simulink model "control_3quads_attached_LIEKF"  (R2019a)
settings: Solver=FixedStepAuto  StartTime=0.0  StopTime=60  FixedStep=0.025  RelTol=1e-3  EnableMultiTasking=on
InitFcn:
  | global clientID;
  | clientID=-1;
  | 
  | global R_t;
  | global A_t;
  | global P_t;
  | global H;
  | global Q;
  | global N;
  | 
  | R_t=eye(3);
  | A_t=eye(3)*0;
  | P_t=eye(3)*0.001;
  | H=eye(3);
  | Q=eye(3);
  | N=eye(3);
values from neighbouring files (symbols this model uses):
  X = reshape(X, size(A_t))    [RiccatiCov.m]
undefined symbols (not defined in the file or in its folder): Y, Z
libraries: robotlib x10, dspindex x3, simulink_extras x1
settings Model: Creator=Kleber Cabral  LastModifiedBy=Kleber Cabral
settings SolverCC: AutoInsertRateTranBlk=on
settings DataIOCC: SaveFormat=Array  ReturnWorkspaceOutputs=off
settings OptimizationCC: LifeSpan=inf
settings DebuggingCC: SolverPrmCheckMsg=warning  SFUnexpectedBacktrackingDiag=warning  SFNoUnconditionalDefaultTransitionDiag=warning  ArithmeticOperatorsInVariantConditions=warning
settings HardwareCC: ProdBitPerPointer=32  ProdBitPerSizeT=32  ProdBitPerPtrDiffT=32  ProdLargestAtomicFloat=None  ProdIntDivRoundTo=Undefined  ProdEndianess=Unspecified  ProdWordSize=32  ProdHWDeviceType=32-bit Generic
settings ModelReferenceCC: PropagateSignalLabelsOutOfModel=off
settings SFSimCC: SimUseLocalCustomCode=off
settings RTWCC: RTWUseLocalCustomCode=off
settings CodeAppCC: StateflowObjectComments=on
settings GRTTargetCC: TargetLangStandard=C89/C90 (ANSI)  GeneratePreprocessorConditionals=Disable all
settings ConfigComp: CovMetricSettings=dw  CovHtmlReporting=on  CovSaveCumulativeToWorkspaceVar=on  CovSaveSingleToWorkspaceVar=on  CovExternalEMLEnable=off  CovSFcnEnable=off

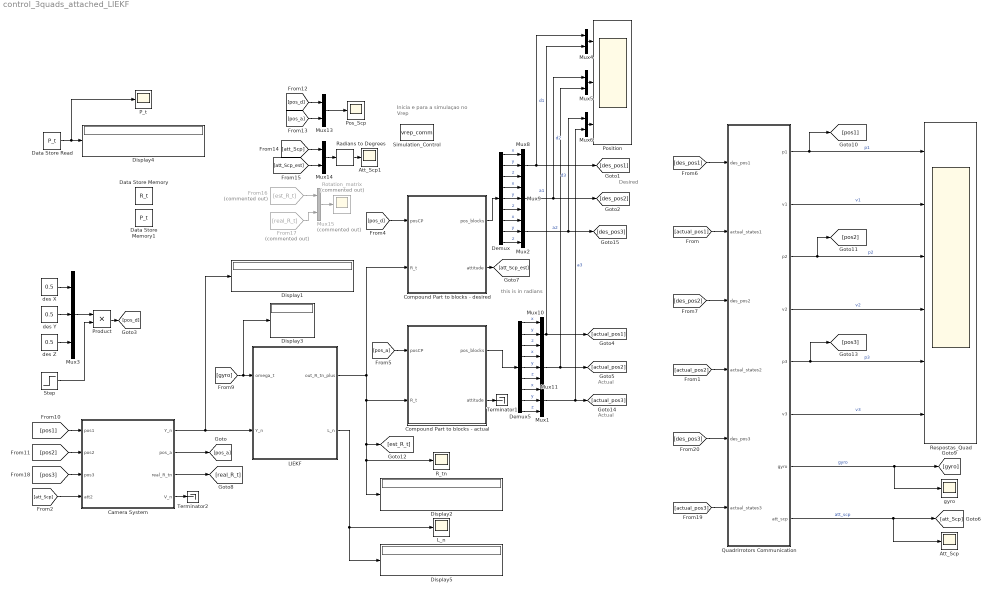
== system control_3quads_attached_LIEKF ==
  note: this is in radians
  note: Desired
  note: Inicia e para a simulaçao no Vrep
  note: Actual
  note: Actual
  Att_Scp : Scope
  Att_Scp1 : Scope
  Camera System : Subsystem
  Compound Part to blocks - actual : MATLAB Function  TreatAsAtomicUnit=on
  Compound Part to blocks - desired : MATLAB Function  TreatAsAtomicUnit=on
  Data Store Memory : DataStoreMemory  DataStoreName=R_t  ReadBeforeWriteMsg=warning  WriteAfterWriteMsg=warning  WriteAfterReadMsg=warning  InitialValue=eye(3)  ShowAdditionalParam=off  OutDataTypeStr=double
  Data Store Memory1 : DataStoreMemory  DataStoreName=P_t  ReadBeforeWriteMsg=warning  WriteAfterWriteMsg=warning  WriteAfterReadMsg=warning  InitialValue=eye(3)*0.001  ShowAdditionalParam=off  OutDataTypeStr=double
  Data Store Read : DataStoreRead  DataStoreName=P_t
  Demux : Demux  Outputs=9
  Demux5 : Demux  Outputs=9
  Display{1..5} (5 alike) : Display
      settings: Decimation=3
  From16 : From  Commented=on  GotoTag=est_R_t
  From17 : From  Commented=on  GotoTag=real_R_t
  LIEKF : MATLAB Function  TreatAsAtomicUnit=on
  L_n : Scope
  Mux{1..3,8..11} (7 alike) : Mux  Inputs=3
  Mux{4..6,13..14} (5 alike) : Mux  Inputs=2
  Mux15 : Mux  Commented=on  Inputs=2
  P_t : Scope
  Pos_Scp : Scope
  Position : Scope  NumInputPorts=3
  Product : Product
  Quadrirrotors Communication : Subsystem
  R_tn : Scope
  Radians to Degrees : simulink_extras/Transformations/Radians to Degrees
  Respostas_Quad : Scope  NumInputPorts=6
  Rotation_matrix : Scope  Commented=on
  Simulation_Control : S-Function  FunctionName=vrep_comm  SFunctionDeploymentMode=off  EnableBusSupport=off
  Step : Step  Time=5  SampleTime=0
  Terminator1 : Terminator
  Terminator2 : Terminator
  des X : Constant  Value=0.5
  des Y : Constant  Value=0.5
  des Z : Constant  Value=0.5
  gyro : Scope
  wires:
  des X/1 -> Mux3/1
  des Y/1 -> Mux3/2
  des Z/1 -> Mux3/3
  [pos1] -> Camera System/1(pos1)
  [pos2] -> Camera System/2(pos2)
  [pos_d] -> Compound Part to blocks - desired/1(posCP)
  Compound Part to blocks - desired/1(pos_blocks) -> Demux/1
  Compound Part to blocks - actual/1(pos_blocks) -> Demux5/1
  Mux8/1 -> Mux4/1, [des_pos1]  "d1"
  Demux/3 -> Mux8/3  "z"
  Demux/2 -> Mux8/2  "y"
  Demux/1 -> Mux8/1  "x"
  Mux9/1 -> Mux5/1, [des_pos2]  "d2"
  Demux/4 -> Mux9/1  "x"
  Demux/5 -> Mux9/2  "y"
  Demux/6 -> Mux9/3  "z"
  [des_pos1] -> Quadrirrotors Communication/1(des_pos1)
  [des_pos2] -> Quadrirrotors Communication/3(des_pos2)
  Mux11/1 -> Mux5/2, [actual_pos2]  "a2"
  Mux10/1 -> Mux4/2, [actual_pos1]  "a1"
  Demux5/1 -> Mux10/1  "x"
  Demux5/2 -> Mux10/2  "y"
  Demux5/3 -> Mux10/3  "z"
  Demux5/4 -> Mux11/1  "x"
  Demux5/5 -> Mux11/2  "y"
  Demux5/6 -> Mux11/3  "z"
  [actual_pos1] -> Quadrirrotors Communication/2(actual_states1)
  [actual_pos2] -> Quadrirrotors Communication/4(actual_states2)
  Camera System/2(pos_a) -> [pos_a]
  [att_Scp] -> Camera System/4(att2)
  Compound Part to blocks - desired/2(attitude) -> [att_Scp_est]
  Camera System/1(Y_n) -> Display1/1, LIEKF/2(Y_n)
  [gyro] -> Display3/1, LIEKF/1(omega_t)
  Compound Part to blocks - actual/2(attitude) -> Terminator1/1
  Data Store Read/1 -> P_t/1, Display4/1
  LIEKF/2(L_n) -> Display5/1, L_n/1
  LIEKF/1(out_R_tn_plus) -> Display2/1, R_tn/1, [est_R_t], Compound Part to blocks - actual/2(R_t), Compound Part to blocks - desired/2(R_t)
  [pos_a] -> Compound Part to blocks - actual/1(posCP)
  Mux3/1 -> Product/1
  Step/1 -> Product/2
  Product/1 -> [pos_d]
  Mux13/1 -> Pos_Scp/1
  [pos_d] -> Mux13/1
  [pos_a] -> Mux13/2
  [att_Scp] -> Mux14/1
  [att_Scp_est] -> Mux14/2
  Camera System/3(real_R_tn) -> [real_R_t]
  Camera System/4(V_n) -> Terminator2/1
  From16/1 -> Mux15/1
  From17/1 -> Mux15/2
  Mux15/1 -> Rotation_matrix/1
  Quadrirrotors Communication/1(p1) -> Respostas_Quad/1, [pos1]  "p1"
  Quadrirrotors Communication/2(v1) -> Respostas_Quad/2  "v1"
  Quadrirrotors Communication/3(p2) -> Respostas_Quad/3, [pos2]  "p2"
  Quadrirrotors Communication/4(v2) -> Respostas_Quad/4  "v2"
  Quadrirrotors Communication/7(gyro) -> gyro/1, [gyro]  "gyro"
  Quadrirrotors Communication/8(att_scp) -> Att_Scp/1, [att_Scp]  "att_scp"
  Quadrirrotors Communication/5(p3) -> Respostas_Quad/5, [pos3]  "p3"
  [pos3] -> Camera System/3(pos3)
  Quadrirrotors Communication/6(v3) -> Respostas_Quad/6  "v3"
  Demux5/9 -> Mux1/3  "z"
  Demux5/8 -> Mux1/2  "y"
  Demux5/7 -> Mux1/1  "x"
  Mux1/1 -> Mux6/2, [actual_pos3]  "a3"
  [actual_pos3] -> Quadrirrotors Communication/6(actual_states3)
  Demux/9 -> Mux2/3  "z"
  Demux/8 -> Mux2/2  "y"
  Demux/7 -> Mux2/1  "x"
  Mux2/1 -> Mux6/1, [des_pos3]  "d3"
  [des_pos3] -> Quadrirrotors Communication/5(des_pos3)
  Mux4/1 -> Position/1
  Mux5/1 -> Position/2
  Mux6/1 -> Position/3
  Radians to Degrees/1 -> Att_Scp1/1
  Mux14/1 -> Radians to Degrees/1

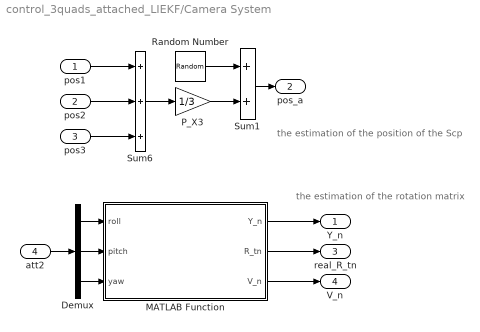
== system control_3quads_attached_LIEKF/Camera System ==
  note: the estimation of the rotation matrix
  note: the estimation of the position of the Scp
  pos1 : Inport
  pos2 : Inport  Port=2
  pos3 : Inport  Port=3
  att2 : Inport  Port=4
  Demux : Demux  Outputs=3
  MATLAB Function : MATLAB Function  TreatAsAtomicUnit=on
  P_X3 : Gain  Gain=1/3
  Random Number : RandomNumber  Variance=0.05
  Sum1 : Sum
  Sum6 : Sum  Inputs=+++
  Y_n : Outport
  pos_a : Outport  Port=2
  real_R_tn : Outport  Port=3
  V_n : Outport  Port=4
  wires:
  pos1/1 -> Sum6/1
  pos2/1 -> Sum6/2
  Sum6/1 -> P_X3/1
  Sum1/1 -> pos_a/1
  att2/1 -> Demux/1
  Demux/3 -> MATLAB Function/3(yaw)
  Demux/2 -> MATLAB Function/2(pitch)
  Demux/1 -> MATLAB Function/1(roll)
  MATLAB Function/1(Y_n) -> Y_n/1
  MATLAB Function/2(R_tn) -> real_R_tn/1
  MATLAB Function/3(V_n) -> V_n/1
  pos3/1 -> Sum6/3
  P_X3/1 -> Sum1/2
  Random Number/1 -> Sum1/1

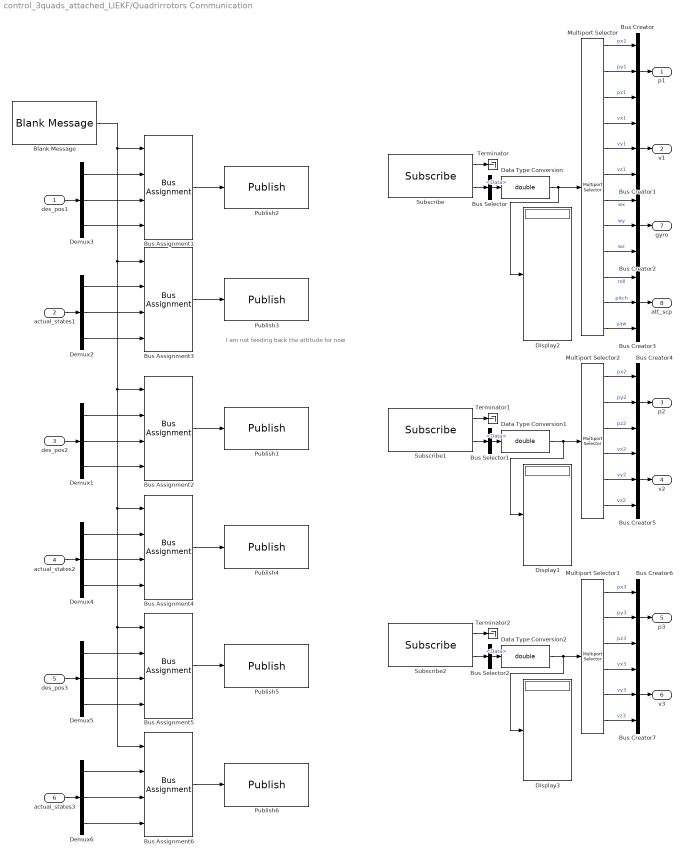
== system control_3quads_attached_LIEKF/Quadrirrotors Communication ==
  note: I am not feeding back the attitude for now
  des_pos1 : Inport
  actual_states1 : Inport  Port=2
  des_pos2 : Inport  Port=3
  actual_states2 : Inport  Port=4
  des_pos3 : Inport  Port=5
  actual_states3 : Inport  Port=6
  Blank Message : robotlib/Blank Message  messageClass=Message  entityType=geometry_msgs/Vector3  messageType=geometry_msgs/Vector3  SampleTime=inf
      settings: SourceProductBaseCode=RO
  Bus Assignment{1..6} (6 alike) : BusAssignment  DialogController=Simulink.DDGSource_BusAssignment  AssignedSignals=X,Y,Z
  Bus Creator{,1..7} (8 alike) : BusCreator  Inputs=3
  Bus Selector : BusSelector  OutputSignals=Data
  Bus Selector1 : BusSelector  OutputSignals=Data
  Bus Selector2 : BusSelector  OutputSignals=Data
  Data Type Conversion : DataTypeConversion  OutDataTypeStr=double
  Data Type Conversion1 : DataTypeConversion  OutDataTypeStr=double
  Data Type Conversion2 : DataTypeConversion  OutDataTypeStr=double
  Demux{1..6} (6 alike) : Demux  Outputs=3
  Display1 : Display
      settings: Decimation=3
  Display2 : Display
      settings: Decimation=3
  Display3 : Display
      settings: Decimation=3
  Multiport Selector : dspindex/Multiport Selector  rowsOrCols=Rows  idxCellArray={1,2,3,4,5,6,7,8,9,10,11,12}  idxErrMode=Clip Index
  Multiport Selector1 : dspindex/Multiport Selector  rowsOrCols=Rows  idxCellArray={1,2,3,4,5,6}  idxErrMode=Clip Index
  Multiport Selector2 : dspindex/Multiport Selector  rowsOrCols=Rows  idxCellArray={1,2,3,4,5,6}  idxErrMode=Clip Index
  Publish1 : robotlib/Publish  topicSource=Select from ROS network  topic=/desired_waypoint_1  messageType=geometry_msgs/Vector3  messageQueueLength=105
      settings: SourceProductBaseCode=RO
  Publish2 : robotlib/Publish  topicSource=Select from ROS network  topic=/desired_waypoint_0  messageType=geometry_msgs/Vector3  messageQueueLength=105
      settings: SourceProductBaseCode=RO
  Publish3 : robotlib/Publish  topicSource=Select from ROS network  topic=/actual_states_0  messageType=geometry_msgs/Vector3  messageQueueLength=105
      settings: SourceProductBaseCode=RO
  Publish4 : robotlib/Publish  topicSource=Select from ROS network  topic=/actual_states_1  messageType=geometry_msgs/Vector3  messageQueueLength=105
      settings: SourceProductBaseCode=RO
  Publish5 : robotlib/Publish  topicSource=Select from ROS network  topic=/desired_waypoint_2  messageType=geometry_msgs/Vector3  messageQueueLength=105
      settings: SourceProductBaseCode=RO
  Publish6 : robotlib/Publish  topicSource=Select from ROS network  topic=/actual_states_2  messageType=geometry_msgs/Vector3  messageQueueLength=105
      settings: SourceProductBaseCode=RO
  Subscribe : robotlib/Subscribe  topicSource=Select from ROS network  topic=/quadrotor_states_0  messageType=std_msgs/Float32MultiArray  sampleTime=-1  messageQueueLength=51
      settings: SourceProductBaseCode=RO
  Subscribe1 : robotlib/Subscribe  topicSource=Select from ROS network  topic=/quadrotor_states_1  messageType=std_msgs/Float32MultiArray  sampleTime=-1  messageQueueLength=51
      settings: SourceProductBaseCode=RO
  Subscribe2 : robotlib/Subscribe  topicSource=Select from ROS network  topic=/quadrotor_states_2  messageType=std_msgs/Float32MultiArray  sampleTime=-1  messageQueueLength=51
      settings: SourceProductBaseCode=RO
  Terminator : Terminator
  Terminator1 : Terminator
  Terminator2 : Terminator
  p1 : Outport
  v1 : Outport  Port=2
  p2 : Outport  Port=3
  v2 : Outport  Port=4
  p3 : Outport  Port=5
  v3 : Outport  Port=6
  gyro : Outport  Port=7
  att_scp : Outport  Port=8
  wires:
  Subscribe/1 -> Terminator/1
  Subscribe/2 -> Bus Selector/1
  Data Type Conversion/1 -> Display2/1, Multiport Selector/1
  Bus Selector/1 -> Data Type Conversion/1  "<Data>"
  Bus Assignment1/1 -> Publish2/1
  Bus Assignment2/1 -> Publish1/1
  Subscribe1/1 -> Terminator1/1
  Subscribe1/2 -> Bus Selector1/1
  Data Type Conversion1/1 -> Display1/1, Multiport Selector2/1
  Bus Selector1/1 -> Data Type Conversion1/1  "<Data>"
  des_pos1/1 -> Demux3/1
  Demux3/1 -> Bus Assignment1/2
  Demux3/2 -> Bus Assignment1/3
  Demux3/3 -> Bus Assignment1/4
  des_pos2/1 -> Demux1/1
  Demux1/1 -> Bus Assignment2/2
  Demux1/2 -> Bus Assignment2/3
  Demux1/3 -> Bus Assignment2/4
  Demux2/3 -> Bus Assignment3/4
  Demux2/2 -> Bus Assignment3/3
  Demux2/1 -> Bus Assignment3/2
  actual_states1/1 -> Demux2/1
  Bus Assignment3/1 -> Publish3/1
  Demux4/3 -> Bus Assignment4/4
  Demux4/2 -> Bus Assignment4/3
  Demux4/1 -> Bus Assignment4/2
  actual_states2/1 -> Demux4/1
  Bus Assignment4/1 -> Publish4/1
  Bus Assignment6/1 -> Publish6/1
  actual_states3/1 -> Demux6/1
  Demux6/1 -> Bus Assignment6/2
  Demux6/2 -> Bus Assignment6/3
  Demux6/3 -> Bus Assignment6/4
  Demux5/3 -> Bus Assignment5/4
  Demux5/2 -> Bus Assignment5/3
  Demux5/1 -> Bus Assignment5/2
  des_pos3/1 -> Demux5/1
  Bus Assignment5/1 -> Publish5/1
  Blank Message/1 -> Bus Assignment3/1, Bus Assignment5/1, Bus Assignment6/1, Bus Assignment4/1, Bus Assignment2/1, Bus Assignment1/1
  Bus Selector2/1 -> Data Type Conversion2/1  "<Data>"
  Data Type Conversion2/1 -> Multiport Selector1/1, Display3/1
  Subscribe2/2 -> Bus Selector2/1
  Subscribe2/1 -> Terminator2/1
  Multiport Selector/3 -> Bus Creator/3  "pz1"
  Multiport Selector/2 -> Bus Creator/2  "py1"
  Bus Creator/1 -> p1/1
  Multiport Selector/6 -> Bus Creator1/3  "vz1"
  Multiport Selector/4 -> Bus Creator1/1  "vx1"
  Multiport Selector/5 -> Bus Creator1/2  "vy1"
  Bus Creator1/1 -> v1/1
  Multiport Selector2/2 -> Bus Creator4/2  "py2"
  Multiport Selector2/3 -> Bus Creator4/3  "pz2"
  Multiport Selector2/1 -> Bus Creator4/1  "px2"
  Bus Creator4/1 -> p2/1
  Multiport Selector2/4 -> Bus Creator5/1  "vx2"
  Multiport Selector2/5 -> Bus Creator5/2  "vy2"
  Multiport Selector2/6 -> Bus Creator5/3  "vz2"
  Bus Creator5/1 -> v2/1
  Bus Creator7/1 -> v3/1
  Multiport Selector1/6 -> Bus Creator7/3  "vz3"
  Multiport Selector1/5 -> Bus Creator7/2  "vy3"
  Multiport Selector1/4 -> Bus Creator7/1  "vx3"
  Bus Creator6/1 -> p3/1
  Multiport Selector1/1 -> Bus Creator6/1  "px3"
  Multiport Selector1/3 -> Bus Creator6/3  "pz3"
  Multiport Selector1/2 -> Bus Creator6/2  "py3"
  Multiport Selector/7 -> Bus Creator2/1  "wx"
  Multiport Selector/8 -> Bus Creator2/2  "wy"
  Multiport Selector/9 -> Bus Creator2/3  "wz"
  Bus Creator2/1 -> gyro/1
  Multiport Selector/10 -> Bus Creator3/1  "roll"
  Multiport Selector/11 -> Bus Creator3/2  "pitch"
  Multiport Selector/12 -> Bus Creator3/3  "yaw"
  Bus Creator3/1 -> att_scp/1
  Multiport Selector/1 -> Bus Creator/1  "px1"

== matlab function control_3quads_attached_LIEKF/LIEKF ==
  data: omega_t input; out_R_tn_plus output; Y_n input; R_t data_store_memory; P_t data_store_memory; L_n output
function [out_R_tn_plus,L_n]  = LIEFK(omega_t,Y_n)

global R_t;
global P_t;

omega_t = omega_t + deg2rad(1)*randn;

disp('>>>>>>>>>>>>>>>>>>>')
%R_t =  reshape(R_t, [3 3]);

% omega_t=u(1:3);
% Y_n = reshape(u(4:12), size(A_t));

%% propagation
%dR_t = R_t * skew_sym(omega_t)
skew_sym_omega=skew_sym_3(omega_t);
[~, X] = ode45(@(t,X)propagation(t, R_t, skew_sym_omega), [0 0.025], R_t);
R_t=reshape(X(size(X,1),:), [3 3]);
R_tn=R_t;

%% update
%FIRST I will compute Ln and P_tn
A_t = - skew_sym_3(omega_t);
H   = eye(3);
Q   = eye(3)*0.1; %covariance of the process noise
N   = eye(3)*0.1; %covariance of the measurement noise

% At this point I will have P_tn-1
%dP_t = A_t * P_t + P_t * (A_t') + Q;
[~, X] = ode45(@(t,X) RiccatiCov (t, P_t, A_t, Q), [0 0.025], P_t);
P_tn=reshape(X(size(X,1),:), size(A_t));
S_n = H * P_tn * (H') + N;
L_n = ( P_tn * (H') ) / S_n; %P_tn * (H') * inv(S_n);
P_tn_plus = (eye(3) - L_n * H) * P_tn;
P_t = P_tn_plus;

% if max(P_t)>0.22
%     pause(0.1)
% end
%Now I update my R_tn
%R_tn_plus = R_tn * exp (Ln * inv (exp(inv(R_tn*Y_n))))
% temp1 = inv(R_tn)
% temp2 = inv(R_tn)*Y_n
% temp3 = expm(inv(R_tn)*Y_n)
% temp4 = inv (expm(inv(R_tn)*Y_n))
% temp5 = L_n * inv (expm(inv(R_tn)*Y_n))
% temp6 = expm (L_n * inv (expm(inv(R_tn)*Y_n)))
% temp7 = R_tn * expm (L_n * inv (expm(inv(R_tn)*Y_n)))
% R_t - R_t * exp (L_n * inv (exp(inv(R_tn)*Y_n)))
% R_t - R_t * exp (L_n * inv (expm(inv(R_tn)*Y_n)))
% R_t - R_t * expm (L_n * inv (exp(inv(R_tn)*Y_n)))
% R_t - R_t * expm (L_n * inv (expm(inv(R_tn)*Y_n)))
% R_tn_plus = R_tn * expm(L_n * inv(expm(inv(R_tn)*Y_n)));
% R_tn_plus = R_tn * expm(L_n /(expm(R_tn\Y_n)));
R_tn_plus = R_tn * expm (L_n *(inv(R_tn)*Y_n- eye(3)));

R_t = R_tn_plus;

%Checking orthogonality of matrix
% R_t' - inv(R_t)

% out_R_tn_plus=[1,2,3;4,5,6;7,8,9];
disp('<<<<<<<<<<<<<<<<<<<<')
out_R_tn_plus=R_tn_plus;
end

== matlab function control_3quads_attached_LIEKF/Camera System/MATLAB Function ==
  data: roll input; Y_n output; pitch input; yaw input; R_tn output; V_n output
function [Y_n,R_tn,V_n] = EulerAng2RotMat(roll, pitch, yaw)
% a=deg2rad(0);
% b=deg2rad(0);
% c=deg2rad(45);

a=roll;
b=pitch;
c=yaw;

sa=sin(a);ca=cos(a);
sb=sin(b);cb=cos(b);
sc=sin(c);cc=cos(c);
R_tn=[ cc*cb cc*sb*sa-sc*ca cc*sb*ca+sc*sa 
    sc*cb sc*sb*sa+cc*ca sc*sb*ca-cc*sa 
    -sb       cb*sa           cb*ca     ];

%noise of about 1 deg of rotation in each axis
a=deg2rad(randn*5);
b=deg2rad(randn*5);
c=deg2rad(randn*5);
sa=sin(a);ca=cos(a);
sb=sin(b);cb=cos(b);
sc=sin(c);cc=cos(c);
V_n=[ cc*cb cc*sb*sa-sc*ca cc*sb*ca+sc*sa 
    sc*cb sc*sb*sa+cc*ca sc*sb*ca-cc*sa 
    -sb       cb*sa           cb*ca     ];

Y_n = R_tn * V_n;

%R = R *(eye(3)+0.001*randn(3,3));
end

== matlab function control_3quads_attached_LIEKF/Compound Part to blocks - actual ==
  data: posCP input; pos_blocks output; R_t input; attitude output
function [ pos_blocks, attitude]  = CP2Blocks(posCP,R_t)
%note that this function works both for desired position of CP and actual
%position CP

%R_t=reshape(R_t, [3 3]);

% positions inside the compound part
d=0.135;
picp = [-d 0 0; 0 0 0; d 0 0];

%% first part, position of each block
s_lb1 = picp(1,:)'; % quadrotor 1
s_lb2 = picp(2,:)'; % quadrotor 2
s_lb3 = picp(3,:)'; % quadrotor 3

s_cp = posCP;

s_b1 = R_t * s_lb1 + s_cp;
s_b2 = R_t * s_lb2 + s_cp;
s_b3 = R_t * s_lb3 + s_cp;

pos_blocks = [s_b1;s_b2;s_b3];

%% Compute the attitude of each block
tform = rotm2tform(R_t);
eul = tform2eul(tform);
attitude = eul;

end

== matlab function control_3quads_attached_LIEKF/Compound Part to blocks - desired ==
  data: posCP input; pos_blocks output; R_t input; attitude output
function [ pos_blocks, attitude ] = CP2Blocks(posCP,R_t)
%note that this function works both for desired position of CP and actual
%position CP

%R_t=reshape(R_t, [3 3]);

% positions inside the compound part
d=0.135;
picp = [-d 0 0; 0 0 0; d 0 0];

%% first part, position of each block
s_lb1 = picp(1,:)'; % quadrotor 1
s_lb2 = picp(2,:)'; % quadrotor 2
s_lb3 = picp(3,:)'; % quadrotor 3

s_cp = posCP;

s_b1 = R_t * s_lb1 + s_cp;
s_b2 = R_t * s_lb2 + s_cp;
s_b3 = R_t * s_lb3 + s_cp;

pos_blocks = [s_b1;s_b2;s_b3];

%% Compute the attitude of each block
tform = rotm2tform(R_t);
eul = tform2eul(tform);
attitude = eul;

end
